simulink model "Prac5_setup"  (R2020b)
settings: Solver=VariableStepAuto  StartTime=0.0  StopTime=10.0  RelTol=1e-3
values from neighbouring files (symbols this model uses):
  a1 = 6.94016215446    [Prac5_paramaters.mat]
  a2 = 6.66666666667    [Prac5_paramaters.mat]
  a5 = 24.7862934088    [Prac5_paramaters.mat]
  a6 = 0.543275668938    [Prac5_paramaters.mat]
  C = 0.97    [prac5_var.m]
  Td = 0.14    [prac5_var.m]
  wn = 4.75    [prac5_var.m]
  zeta = 0.081    [prac5_var.m]
undefined symbols (not defined in the file or in its folder): cputime
settings Model: Creator=mluser  LastModifiedBy=mluser

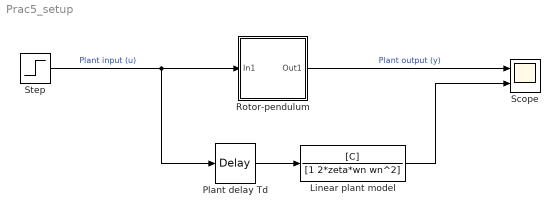
== system Prac5_setup ==
  Linear plant model : TransferFcn  Numerator=[C]  Denominator=[1 2*zeta*wn wn^2]
  Plant delay Td : TransportDelay  DelayTime=Td
  Rotor-pendulum : Subsystem  Description=Rotor pendulum
  Scope : Scope  NumInputPorts=2
  Step : Step  After=10  SampleTime=0
  wires:
  Step/1 -> Plant delay Td/1, Rotor-pendulum/1(In1)  "Plant input (u)"
  Rotor-pendulum/1(Out1) -> Scope/1  "Plant output (y)"
  Plant delay Td/1 -> Linear plant model/1
  Linear plant model/1 -> Scope/2

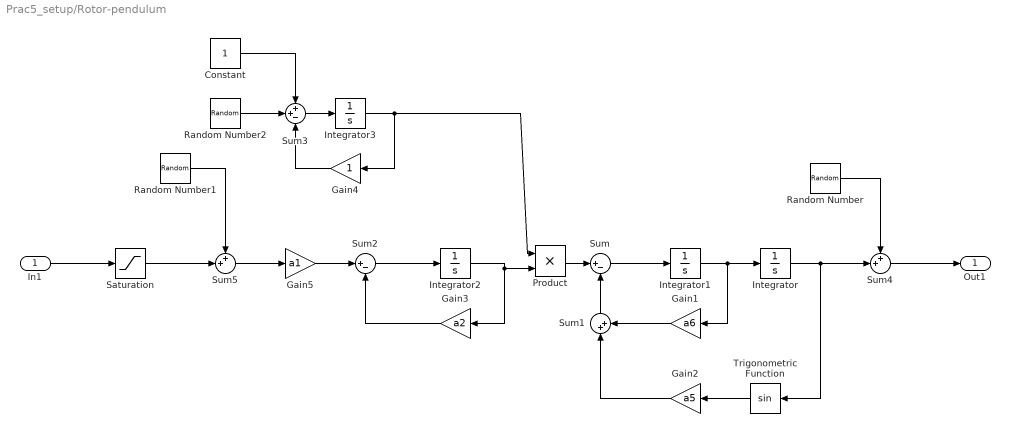
== system Prac5_setup/Rotor-pendulum ==
  In1 : Inport
  Constant : Constant
  Gain1 : Gain  Gain=a6
  Gain2 : Gain  Gain=a5
  Gain3 : Gain  Gain=a2
  Gain4 : Gain
  Gain5 : Gain  Gain=a1
  Integrator : Integrator
  Integrator1 : Integrator
  Integrator2 : Integrator
  Integrator3 : Integrator  InitialCondition=1
  Product : Product
  Random Number : RandomNumber  Variance=0.005^2  Seed=round(cputime*100)  SampleTime=0.001
  Random Number1 : RandomNumber  Variance=0.5^2  Seed=round(cputime*100)  SampleTime=0.001
  Random Number2 : RandomNumber  Variance=0.5^2  Seed=round(cputime*100)  SampleTime=0.001
  Saturation : Saturate  UpperLimit=15  LowerLimit=-15
  Sum : Sum  Inputs=|+-
  Sum1 : Sum  Inputs=|++
  Sum2 : Sum  Inputs=|+-
  Sum3 : Sum  Inputs=++-
  Sum4 : Sum  Inputs=++|
  Sum5 : Sum  Inputs=++|
  Trigonometric Function : Trigonometry
  Out1 : Outport
  wires:
  Gain2/1 -> Sum1/1
  Integrator1/1 -> Gain1/1, Integrator/1
  Sum1/1 -> Sum/2
  Gain5/1 -> Sum2/1
  Random Number1/1 -> Sum5/1
  Sum/1 -> Integrator1/1
  Sum2/1 -> Integrator2/1
  Sum5/1 -> Gain5/1
  Integrator2/1 -> Product/2, Gain3/1
  Sum4/1 -> Out1/1
  Gain1/1 -> Sum1/2
  Integrator/1 -> Sum4/2, Trigonometric Function/1
  Random Number/1 -> Sum4/1
  Trigonometric Function/1 -> Gain2/1
  Gain3/1 -> Sum2/2
  In1/1 -> Saturation/1
  Saturation/1 -> Sum5/2
  Sum3/1 -> Integrator3/1
  Product/1 -> Sum/1
  Integrator3/1 -> Gain4/1, Product/1
  Random Number2/1 -> Sum3/2
  Gain4/1 -> Sum3/3
  Constant/1 -> Sum3/1
